simulink model "Subsystem0"  (R2020b)
settings: Solver=FixedStepAuto  StartTime=0.0  StopTime=10.0  FixedStep=0.2  RelTol=1e-3
settings Model: Creator=nadee  LastModifiedBy=nadee
settings DataIOCC: SaveOutput=off  SaveTime=off

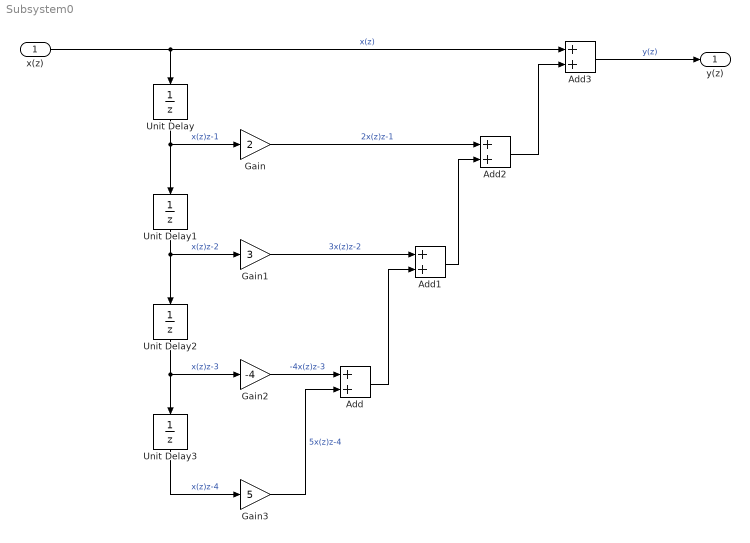
== system Subsystem0 ==
  x(z) : Inport  OutDataTypeStr=double  PortDimensions=1  SampleTime=[0.20000000000000001,0]
  Add{,1..3} (4 alike) : Sum
  Gain : Gain  Gain=2
  Gain1 : Gain  Gain=3
  Gain2 : Gain  Gain=-4
  Gain3 : Gain  Gain=5
  Unit Delay{,1..3} (4 alike) : UnitDelay  SampleTime=-1  HasFrameUpgradeWarning=on
  y(z) : Outport  OutDataTypeStr=double  PortDimensions=1  SampleTime=[0.20000000000000001,0]
  wires:
  Unit Delay3/1 -> Gain3/1  "x(z)z-4"
  Unit Delay1/1 -> Gain1/1, Unit Delay2/1  "x(z)z-2"
  Add1/1 -> Add2/2
  x(z)/1 -> Add3/1, Unit Delay/1  "x(z)"
  Unit Delay2/1 -> Unit Delay3/1, Gain2/1  "x(z)z-3"
  Unit Delay/1 -> Unit Delay1/1, Gain/1  "x(z)z-1"
  Add3/1 -> y(z)/1  "y(z)"
  Add2/1 -> Add3/2
  Add/1 -> Add1/2
  Gain/1 -> Add2/1  "2x(z)z-1"
  Gain2/1 -> Add/1  "-4x(z)z-3"
  Gain1/1 -> Add1/1  "3x(z)z-2"
  Gain3/1 -> Add/2  "5x(z)z-4"
